simulink model "Battery_charge_discharge_FSBB_DCDC_r2020_batterySelfDesigned"  (R2020a)
settings: Solver=ode23tb  StartTime=0.0  StopTime=1  MaxStep=2.2222222222222224E-7  RelTol=1e-3  EnableMultiTasking=on
undefined symbols (not defined in the file or in its folder): Ion, Lithium, sigbuilder_block
libraries: powerlib x175, dsparch4 x4, simulink x4, electricdrivelib x1, powerlib_meascontrol x1
(part 1 of 2)
settings Model: Creator=Lei  LastModifiedBy=Loki
settings DataIOCC: LimitDataPoints=on  SaveFormat=Array  ReturnWorkspaceOutputs=off
settings OptimizationCC: LifeSpan=inf
settings DebuggingCC: SolverPrmCheckMsg=warning  SFUnexpectedBacktrackingDiag=warning  SFNoUnconditionalDefaultTransitionDiag=warning  SFExecutionAtInitializationDiag=none  ArithmeticOperatorsInVariantConditions=warning
settings HardwareCC: ProdBitPerPointer=32  ProdBitPerSizeT=32  ProdBitPerPtrDiffT=32  ProdLargestAtomicFloat=None  ProdIntDivRoundTo=Undefined  ProdEndianess=Unspecified  ProdWordSize=32  ProdHWDeviceType=32-bit Generic
settings ModelReferenceCC: PropagateSignalLabelsOutOfModel=off
settings SFSimCC: SimUseLocalCustomCode=off  CustomCodeUndefinedFunction=UseInterfaceOnly
settings RTWCC: RTWUseLocalCustomCode=off
settings CodeAppCC: StateflowObjectComments=on
settings GRTTargetCC: TargetLangStandard=C89/C90 (ANSI)
settings ConfigComp: CovMetricSettings=dw  CovSaveCumulativeToWorkspaceVar=on  CovSaveSingleToWorkspaceVar=on  CovExternalEMLEnable=off  CovSFcnEnable=off
settings SimscapeCC: SimscapeNormalizeSystem=off

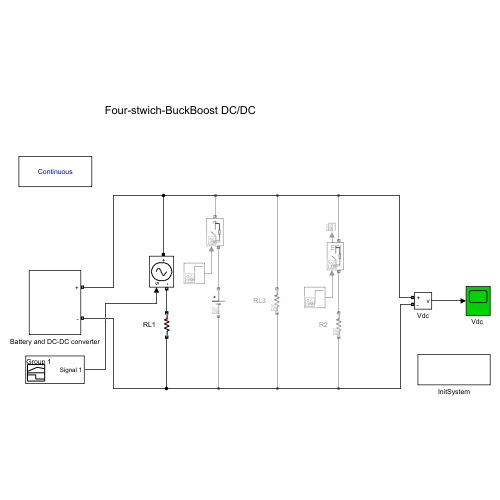
[thumbnail: Simulink's stored preview of the top-level diagram]
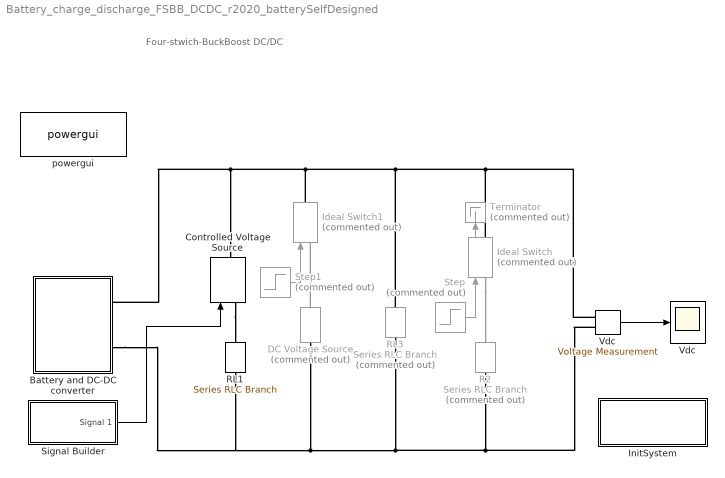
== system Battery_charge_discharge_FSBB_DCDC_r2020_batterySelfDesigned ==
  note: Four-stwich-BuckBoost DC/DC
  Battery and DC-DC converter : Subsystem
  Controlled Voltage Source : powerlib/Electrical Sources/Controlled Voltage Source  Initialize=on  Source_Type=DC  Amplitude=98  Phase=0  Frequency=0  Measurements=None
  DC Voltage Source : powerlib/Electrical Sources/DC Voltage Source  Commented=on  Amplitude=96  Measurements=None
  Ideal Switch : powerlib/Power Electronics/Ideal Switch  Commented=on  Ron=0.001  Lon=0  IC=0  Rs=1e5  Cs=inf  Measurements=on
  Ideal Switch1 : powerlib/Power Electronics/Ideal Switch  Commented=on  Ron=0.001  Lon=0  IC=0  Rs=1e5  Cs=inf  Measurements=off
  InitSystem : Subsystem
      settings: OpenFcn=Battery_charge_discharge_FSBB_param_init
  R2 : powerlib/Elements/Series RLC Branch  Commented=on  LConnTagsString=__new0  RConnTagsString=__new0  BranchType=R  Resistance=6  Inductance=1e-3  SetiL0=off  InitialCurrent=0  Capacitance=1e-6  Setx0=off  InitialVoltage=0  Measurements=None
  RL1 : powerlib/Elements/Series RLC Branch  LConnTagsString=__new0  RConnTagsString=__new0  BranchType=R  Resistance=0.01  Inductance=1e-3  SetiL0=off  InitialCurrent=0  Capacitance=1e-6  Setx0=off  InitialVoltage=0  Measurements=None
  RL3 : powerlib/Elements/Series RLC Branch  Commented=on  LConnTagsString=__new0  RConnTagsString=__new0  BranchType=R  Resistance=3  Inductance=1e-3  SetiL0=off  InitialCurrent=0  Capacitance=1e-6  Setx0=off  InitialVoltage=0  Measurements=None
  Signal Builder : Subsystem  Tag=STV Subsys  LoadFcn=sigbuilder_block('load');  StartFcn=sigbuilder_block('start');  StopFcn=sigbuilder_block('stop');  ClipboardFcn=sigbuilder_block('clipboard');  mask(Sigbuilder block){tuvar=[0:10]}
      mask help: Simulink:masks:SigbuilderBlock_MD
      mask init:
      | if ~strcmp(get_param(bdroot(gcbh),'SimulationStatus'),'stopped') tuvar = sigbuilder_block('maskInit'); end
      settings: CopyFcn=sigbuilder_block('copy');  DeleteFcn=sigbuilder_block('delete');  ModelCloseFcn=sigbuilder_block('modelClose');  PreSaveFcn=sigbuilder_block('preSave');  PauseFcn=sigbuilder_block('pause');  ContinueFcn=sigbuilder_block('continue');  NameChangeFcn=sigbuilder_block('namechange');  OpenFcn=sigbuilder_block('open',[5.4 7.2 1141.2 492.6 ]);  CloseFcn=sigbuilder_block('close');
      mask Display: plot(0, 0, 100, 100,[2, 2, 32, 32, 2], [68, 8, 8, 68, 68],[32, 2], [38, 38], [32, 19, 2],[53, 60, 44], [32, 17, 17, 2],[16, 16, 31, 31]);txt = getActiveGroup(gcbh);text(2, 100, txt,'verticalAlignment', 'top');
  Step : Step  Commented=on  Time=0.3  After=3  SampleTime=0
  Step1 : Step  Commented=on  Time=0.2  SampleTime=0
  Terminator : Terminator  Commented=on
  Vdc : powerlib/Measurements/Voltage Measurement  PhasorSimulation=off  OutputType=Complex  PSBequivalent=0
  "Vdc " : Scope
  powergui : powerlib/powergui  Priority=1  SimulationMode=Continuous  SampleTime=1/45000/100  frequency=60  Iterations=50  frequencyindice=0  Pbase=100e6  ErrMax=1e-4  UnitsV=kV  UnitsW=MW  buscounter=0  FunctionMessages=off  echomessages=off  EnableUseOfTLC=off  CurrentSourceSwitches=off  DisableSnubberDevices=off  DisableRonSwitches=off  DisableVfSwitches=off  DisplayEquations=off  AutomaticDiscreteSolvers=off  SolverType=Tustin/Backward Euler (TBE)  Interpol=off  ExternalGateDelay=off  methode=off  Ts=100  x0status=blocks  SPID=off  SwTol=0  HookPort=off  NonlinearTolerance=1e-4  nMaxIteration=100  ContinueOnMaxIteration=off  RestoreLinks=warning  ResistiveCurrentMeasurement=off  Frange=[0:2:500]  Ylog=off  Xlog=on  ShowGrid=off  save=off  variable=ZData  structure=0  ZoomFFT=off  StartTime=0.0  cycles=1  DisplayStyle=1  fundamental=60  FreqAxis=off  MaxFrequency=1000  frequencyindicesteady=1  RmsSteady=1  display=off
  wires:
  Vdc/1 -> "Vdc "/1
  Step/1 -> Ideal Switch/1
  Ideal Switch/1 -> Terminator/1
  Signal Builder/1(Signal 1) -> Controlled Voltage Source/1
  Step1/1 -> Ideal Switch1/1
  connections:
  Vdc/LConn1 -- Ideal Switch/RConn1 -- Ideal Switch1/RConn1 -- Controlled Voltage Source/RConn1 -- Battery and DC-DC converter/RConn1 -- RL3/LConn1
  Ideal Switch/LConn1 -- R2/LConn1
  Vdc/LConn2 -- R2/RConn1 -- RL1/RConn1 -- Battery and DC-DC converter/RConn2 -- DC Voltage Source/LConn1 -- RL3/RConn1
  Controlled Voltage Source/LConn1 -- RL1/LConn1
  DC Voltage Source/RConn1 -- Ideal Switch1/LConn1

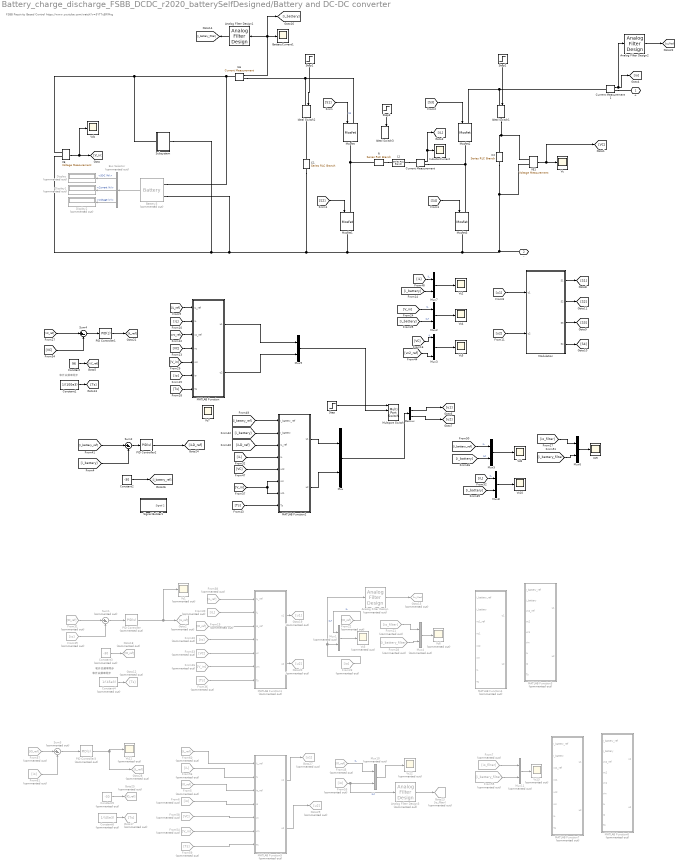
== system Battery_charge_discharge_FSBB_DCDC_r2020_batterySelfDesigned/Battery and DC-DC converter ==
  note: 和开关频率同步
  note: FSBB Passivity Based Control
      | https://www.youtube.com/watch?v=5YT7cERlMrg
  note: 和开关频率同步
  note: 和开关频率同步
  Analog Filter Design : dsparch4/Analog Filter Design  Commented=on  method=Butterworth  filttype=Lowpass  N=1  Wlo=1000  Whi=80  Rp=2  Rs=40
  Analog Filter Design1 : dsparch4/Analog Filter Design  method=Butterworth  filttype=Lowpass  N=1  Wlo=1000  Whi=80  Rp=2  Rs=40
  Analog Filter Design2 : dsparch4/Analog Filter Design  method=Butterworth  filttype=Lowpass  N=1  Wlo=1000  Whi=80  Rp=2  Rs=40
  Analog Filter Design3 : dsparch4/Analog Filter Design  Commented=on  method=Butterworth  filttype=Lowpass  N=1  Wlo=1000  Whi=80  Rp=2  Rs=40
  Battery3 : electricdrivelib/Extra Sources/Battery  Commented=on  BatType=Lithium-Ion  ShowTempParam=off  ThermalPreset=no  ShowAgeParam=off  NomV=102.5  NomQ=10  SOC=50  Batt_Tr=1  PresetModel=on  MaxQ=10  MinV=76.875  FullV=119.3087  Dis_rate=4.3478  R=0.1025  Normal_OP=9.0435  expZone="[110.7395     0.4913043]"  current=[6.5 13 32.5]  Units=Time  Tci=20  NomT=20  T2=-30  MaxQ2=4.8  FullV2=7.1  Normal_OP2=5.655  expZone2="[6.58           1]"  Rca=0.6  ti=2000  Dp=0  Neq0=0  Tsim=1e6  Ta1=25  Qeol=5.4*0.9  Reol=0.013333*1.2  Char_age=[2.3478, 3]  Dis_age=[2.3478, 10]  N1=1500  N2=10500  N3=1000  N4=1400  Ta2=45  N5=950
  BatteryCurrent1 : Scope
  Bus Selector : BusSelector  Commented=on  OutputSignals=SOC (%),Current (A),Voltage (V)
  C1 : powerlib/Elements/Series RLC Branch  LConnTagsString=__new0  RConnTagsString=__new0  BranchType=RC  Resistance=0.001  Inductance=1e-3  SetiL0=off  InitialCurrent=0  Capacitance=1440e-6  Setx0=off  InitialVoltage=80  Measurements=None
  C2 : powerlib/Elements/Series RLC Branch  LConnTagsString=__new0  RConnTagsString=__new0  BranchType=RC  Resistance=0.001  Inductance=1e-3  SetiL0=off  InitialCurrent=0  Capacitance=1440e-6  Setx0=off  InitialVoltage=80  Measurements=None
  Constant : Constant  Value=96
  Constant1 : Constant  Value=1/(100e3)
  Constant2 : Constant  Value=-30
  Constant3 : Constant  Commented=on  Value=-30
  Constant4 : Constant  Commented=on  Value=1/(45e3)
  Constant5 : Constant  Commented=on  Value=-30
  Constant6 : Constant  Commented=on  Value=1/(45e3)
  Current Measurement : powerlib/Measurements/Current Measurement  PhasorSimulation=off  OutputType=Complex  PSBequivalent=0
  Current Measurement1 : powerlib/Measurements/Current Measurement  PhasorSimulation=off  OutputType=Complex  PSBequivalent=0
  Demux : Demux  Outputs=2
  Display : Display  Commented=on
  Display1 : Display  Commented=on
  Display2 : Display  Commented=on
  From{5,19,22,31,45,57} (6 alike) : From  Commented=on  GotoTag=IO_ref
  From{6,20,23,39,53,61} (6 alike) : From  Commented=on  GotoTag=io
  From21 : From  Commented=on  GotoTag=io_filter
  From26 : From  Commented=on  GotoTag=V_in
  From28 : From  Commented=on  GotoTag=i_battery_filter
  From30 : From  Commented=on  GotoTag=iL
  From33 : From  Commented=on  GotoTag=VC
  From36 : From  Commented=on  GotoTag=Ts
  From38 : From  Commented=on  GotoTag=iL_ref
  From54 : From  Commented=on  GotoTag=V_in
  From55 : From  Commented=on  GotoTag=i_battery_filter
  From56 : From  Commented=on  GotoTag=iL
  From58 : From  Commented=on  GotoTag=VC
  From59 : From  Commented=on  GotoTag=Ts
  From60 : From  Commented=on  GotoTag=iL_ref
  From7 : From  Commented=on  GotoTag=io_filter
  Goto12 : Goto  Commented=on  GotoTag=Ts
  Goto15 : Goto  Commented=on  GotoTag=io_filter
  Goto17 : Goto  Commented=on  GotoTag=Ts
  Goto18 : Goto  Commented=on  GotoTag=IO_ref
  Goto19 : Goto  Commented=on  GotoTag=u1
  Goto2 : Goto  Commented=on  GotoTag=iL_ref
  Goto20 : Goto  Commented=on  GotoTag=u2
  Goto23 : Goto  Commented=on  GotoTag=io_filter
  Goto25 : Goto  Commented=on  GotoTag=IO_ref
  Goto27 : Goto  Commented=on  GotoTag=u1
  Goto28 : Goto  Commented=on  GotoTag=iL_ref
  Goto29 : Goto  Commented=on  GotoTag=u2
  IL6 : powerlib/Measurements/Current Measurement  PhasorSimulation=off  OutputType=Complex  PSBequivalent=0
  Ideal Switch1 : powerlib/Power Electronics/Ideal Switch  Ron=1e-6  Lon=0  IC=0  Rs=3  Cs=inf  Measurements=off
  Ideal Switch2 : powerlib/Power Electronics/Ideal Switch  Ron=1e-6  Lon=0  IC=0  Rs=3  Cs=inf  Measurements=off
  Ideal Switch3 : powerlib/Power Electronics/Ideal Switch  Ron=1e-6  Lon=0  IC=0  Rs=3  Cs=inf  Measurements=on
  InductorCurrent : Scope
  L1 : powerlib/Elements/Series RLC Branch  LConnTagsString=__new0  RConnTagsString=__new0  BranchType=L  Resistance=1.0  Inductance=20e-6  SetiL0=off  InitialCurrent=0  Capacitance=1.0  Setx0=off  InitialVoltage=0  Measurements=None
  MATLAB Function : MATLAB Function  TreatAsAtomicUnit=on
  MATLAB Function1 : MATLAB Function  Commented=on  TreatAsAtomicUnit=on
  MATLAB Function2 : MATLAB Function  TreatAsAtomicUnit=on
  MATLAB Function3 : MATLAB Function  Commented=on  TreatAsAtomicUnit=on
  MATLAB Function4 : MATLAB Function  Commented=on  TreatAsAtomicUnit=on
  MATLAB Function5 : MATLAB Function  Commented=on  TreatAsAtomicUnit=on
  MATLAB Function6 : MATLAB Function  Commented=on  TreatAsAtomicUnit=on
  MATLAB Function7 : MATLAB Function  Commented=on  TreatAsAtomicUnit=on
  Modulation : Subsystem
  Mosfet{,1..3} (4 alike) : powerlib/Power Electronics/Mosfet  Ron=0.1  Lon=0  Rd=0.01  Vfd=0  IC=0  Rs=1e5  Cs=inf  Measurements=off
  Multiport Switch : MultiPortSwitch
  Mux{,2,5..9} (7 alike) : Mux  Inputs=2
  Mux{1,4,10..11} (4 alike) : Mux  Commented=on  Inputs=2
  Mux3 : Mux  Inputs=3
  PID Controller : simulink/Continuous/PID Controller  Commented=on  Controller=PID  Form=Parallel  TimeDomain=Continuous-time  UseExternalTs=off  SampleTime=-1  IntegratorMethod=Forward Euler  FilterMethod=Forward Euler  ControllerParametersSource=internal  P=15  I=1000  D=0  N=100  UseFilter=on  TunerSelectOption=Transfer Function Based (PID Tuner App)  InitialConditionSource=internal  InitialConditionForIntegrator=0  InitialConditionForFilter=0  DifferentiatorICPrevScaledInput=0  ExternalReset=none  TrackingMode=off  Kt=1  LimitOutput=off  UpperSaturationLimit=inf  LowerSaturationLimit=-inf  LinearizeAsGain=on  AntiWindupMode=none  Kb=1  POutMin=[]  POutMax=[]  IOutMin=[]  IOutMax=[]  DOutMin=[]  DOutMax=[]  NOutMin=[]  NOutMax=[]  SumOutMin=[]  SumOutMax=[]  SaturationOutMin=[]  SaturationOutMax=[]  PParamMin=[]  PParamMax=[]  IParamMin=[]  IParamMax=[]  DParamMin=[]  DParamMax=[]  NParamMin=[]  NParamMax=[]  KbParamMin=[]  KbParamMax=[]  KtParamMin=[]  KtParamMax=[]  KbOutMin=[]  KbOutMax=[]  KtOutMin=[]  KtOutMax=[]  IntegratorOutMin=[]  IntegratorOutMax=[]  FilterOutMin=[]  FilterOutMax=[]  SumI1OutMin=[]  SumI1OutMax=[]  SumI2OutMin=[]  SumI2OutMax=[]  SumI3OutMin=[]  SumI3OutMax=[]  SumI4OutMin=[]  SumI4OutMax=[]  SumDOutMin=[]  SumDOutMax=[]  DifferentiatorOutMin=[]  DifferentiatorOutMax=[]  FilterDiffOutCoefMin=[]  FilterDiffOutCoefMax=[]  ReciprocalOutMin=[]  ReciprocalOutMax=[]  SumDenOutMin=[]  SumDenOutMax=[]  SumNumOutMin=[]  SumNumOutMax=[]  DivideOutMin=[]  DivideOutMax=[]  UdiffTsProdOutMin=[]  UdiffTsProdOutMax=[]  NTsProdOutMin=[]  NTsProdOutMax=[]  UintegralTsProdOutMin=[]  UintegralTsProdOutMax=[]  UngainTsProdOutMin=[]  UngainTsProdOutMax=[]  IntegratorContinuousStateAttributes=''  IntegratorStateMustResolveToSignalObject=off  IntegratorRTWStateStorageClass=Auto  FilterContinuousStateAttributes=''  FilterStateMustResolveToSignalObject=off  FilterRTWStateStorageClass=Auto  ParallelPVariant=InternalParameters  IdealPVariant=Disabled  IVariant=InternalParameters  DVariant=InternalParameters  IntegratorVariant=Continuous  SatVariant=Disabled  AWVariant=Passthrough  PCopyVariant=Disabled  TRVariant=Disabled  FdbkBlocksVariant=Forward  IdealPFdbkVariant=Disabled  SatFdbkVariant=Disabled  DerivativeFilterVariant=ContFilter  NVariant=InternalParameters  NCopyVariant=Disabled  FilterICVariant=InternalICsFilter  IntegratorICVariant=InternalICs  ExternalResetVariant=Disabled  TRSumVariant=Passthrough  SumFdbkVariant=Disabled  SumVariant=Sum_PID  TsampFilterVariant=InternalTs  TsampNgainVariant=Passthrough  TsampIntegralVariant=Passthrough
  PID Controller1 : simulink/Continuous/PID Controller  Controller=PID  Form=Parallel  TimeDomain=Discrete-time  UseExternalTs=off  SampleTime=-1  IntegratorMethod=Forward Euler  FilterMethod=Forward Euler  ControllerParametersSource=internal  P=15  I=1000  D=0  N=100  UseFilter=on  TunerSelectOption=Transfer Function Based (PID Tuner App)  InitialConditionSource=internal  InitialConditionForIntegrator=0  InitialConditionForFilter=0  DifferentiatorICPrevScaledInput=0  ExternalReset=none  TrackingMode=off  Kt=1  LimitOutput=off  UpperSaturationLimit=inf  LowerSaturationLimit=-inf  LinearizeAsGain=on  AntiWindupMode=none  Kb=1  POutMin=[]  POutMax=[]  IOutMin=[]  IOutMax=[]  DOutMin=[]  DOutMax=[]  NOutMin=[]  NOutMax=[]  SumOutMin=[]  SumOutMax=[]  SaturationOutMin=[]  SaturationOutMax=[]  PParamMin=[]  PParamMax=[]  IParamMin=[]  IParamMax=[]  DParamMin=[]  DParamMax=[]  NParamMin=[]  NParamMax=[]  KbParamMin=[]  KbParamMax=[]  KtParamMin=[]  KtParamMax=[]  KbOutMin=[]  KbOutMax=[]  KtOutMin=[]  KtOutMax=[]  IntegratorOutMin=[]  IntegratorOutMax=[]  FilterOutMin=[]  FilterOutMax=[]  SumI1OutMin=[]  SumI1OutMax=[]  SumI2OutMin=[]  SumI2OutMax=[]  SumI3OutMin=[]  SumI3OutMax=[]  SumI4OutMin=[]  SumI4OutMax=[]  SumDOutMin=[]  SumDOutMax=[]  DifferentiatorOutMin=[]  DifferentiatorOutMax=[]  FilterDiffOutCoefMin=[]  FilterDiffOutCoefMax=[]  ReciprocalOutMin=[]  ReciprocalOutMax=[]  SumDenOutMin=[]  SumDenOutMax=[]  SumNumOutMin=[]  SumNumOutMax=[]  DivideOutMin=[]  DivideOutMax=[]  UdiffTsProdOutMin=[]  UdiffTsProdOutMax=[]  NTsProdOutMin=[]  NTsProdOutMax=[]  UintegralTsProdOutMin=[]  UintegralTsProdOutMax=[]  UngainTsProdOutMin=[]  UngainTsProdOutMax=[]  IntegratorContinuousStateAttributes=''  IntegratorStateMustResolveToSignalObject=off  IntegratorRTWStateStorageClass=Auto  FilterContinuousStateAttributes=''  FilterStateMustResolveToSignalObject=off  FilterRTWStateStorageClass=Auto  ParallelPVariant=InternalParameters  IdealPVariant=Disabled  IVariant=InternalParameters  DVariant=InternalParameters  IntegratorVariant=Discrete  SatVariant=Disabled  AWVariant=Passthrough  PCopyVariant=Disabled  TRVariant=Disabled  FdbkBlocksVariant=Forward  IdealPFdbkVariant=Disabled  SatFdbkVariant=Disabled  DerivativeFilterVariant=ForwardEulerFilter  NVariant=InternalParameters  NCopyVariant=Disabled  FilterICVariant=InternalICsFilter  IntegratorICVariant=InternalICs  ExternalResetVariant=Disabled  TRSumVariant=Passthrough  SumFdbkVariant=Disabled  SumVariant=Sum_PID  TsampFilterVariant=InternalTs  TsampNgainVariant=Passthrough  TsampIntegralVariant=Passthrough
  PID Controller2 : simulink/Continuous/PID Controller  Controller=PID  Form=Parallel  TimeDomain=Continuous-time  UseExternalTs=off  SampleTime=-1  IntegratorMethod=Forward Euler  FilterMethod=Forward Euler  ControllerParametersSource=internal  P=15  I=2000  D=0  N=100  UseFilter=on  TunerSelectOption=Transfer Function Based (PID Tuner App)  InitialConditionSource=internal  InitialConditionForIntegrator=0  InitialConditionForFilter=0  DifferentiatorICPrevScaledInput=0  ExternalReset=none  TrackingMode=off  Kt=1  LimitOutput=off  UpperSaturationLimit=100  LowerSaturationLimit=-100  LinearizeAsGain=off  AntiWindupMode=none  Kb=1  POutMin=[]  POutMax=[]  IOutMin=[]  IOutMax=[]  DOutMin=[]  DOutMax=[]  NOutMin=[]  NOutMax=[]  SumOutMin=[]  SumOutMax=[]  SaturationOutMin=[]  SaturationOutMax=[]  PParamMin=[]  PParamMax=[]  IParamMin=[]  IParamMax=[]  DParamMin=[]  DParamMax=[]  NParamMin=[]  NParamMax=[]  KbParamMin=[]  KbParamMax=[]  KtParamMin=[]  KtParamMax=[]  KbOutMin=[]  KbOutMax=[]  KtOutMin=[]  KtOutMax=[]  IntegratorOutMin=[]  IntegratorOutMax=[]  FilterOutMin=[]  FilterOutMax=[]  SumI1OutMin=[]  SumI1OutMax=[]  SumI2OutMin=[]  SumI2OutMax=[]  SumI3OutMin=[]  SumI3OutMax=[]  SumI4OutMin=[]  SumI4OutMax=[]  SumDOutMin=[]  SumDOutMax=[]  DifferentiatorOutMin=[]  DifferentiatorOutMax=[]  FilterDiffOutCoefMin=[]  FilterDiffOutCoefMax=[]  ReciprocalOutMin=[]  ReciprocalOutMax=[]  SumDenOutMin=[]  SumDenOutMax=[]  SumNumOutMin=[]  SumNumOutMax=[]  DivideOutMin=[]  DivideOutMax=[]  UdiffTsProdOutMin=[]  UdiffTsProdOutMax=[]  NTsProdOutMin=[]  NTsProdOutMax=[]  UintegralTsProdOutMin=[]  UintegralTsProdOutMax=[]  UngainTsProdOutMin=[]  UngainTsProdOutMax=[]  IntegratorContinuousStateAttributes=''  IntegratorStateMustResolveToSignalObject=off  IntegratorRTWStateStorageClass=Auto  FilterContinuousStateAttributes=''  FilterStateMustResolveToSignalObject=off  FilterRTWStateStorageClass=Auto  ParallelPVariant=InternalParameters  IdealPVariant=Disabled  IVariant=InternalParameters  DVariant=InternalParameters  IntegratorVariant=Continuous  SatVariant=Disabled  AWVariant=Passthrough  PCopyVariant=Disabled  TRVariant=Disabled  FdbkBlocksVariant=Forward  IdealPFdbkVariant=Disabled  SatFdbkVariant=Disabled  DerivativeFilterVariant=ContFilter  NVariant=InternalParameters  NCopyVariant=Disabled  FilterICVariant=InternalICsFilter  IntegratorICVariant=InternalICs  ExternalResetVariant=Disabled  TRSumVariant=Passthrough  SumFdbkVariant=Disabled  SumVariant=Sum_PID  TsampFilterVariant=InternalTs  TsampNgainVariant=Passthrough  TsampIntegralVariant=Passthrough
  PID Controller3 : simulink/Continuous/PID Controller  Commented=on  Controller=PID  Form=Parallel  TimeDomain=Continuous-time  UseExternalTs=off  SampleTime=-1  IntegratorMethod=Forward Euler  FilterMethod=Forward Euler  ControllerParametersSource=internal  P=15  I=1000  D=0  N=100  UseFilter=on  TunerSelectOption=Transfer Function Based (PID Tuner App)  InitialConditionSource=internal  InitialConditionForIntegrator=0  InitialConditionForFilter=0  DifferentiatorICPrevScaledInput=0  ExternalReset=none  TrackingMode=off  Kt=1  LimitOutput=off  UpperSaturationLimit=inf  LowerSaturationLimit=-inf  LinearizeAsGain=on  AntiWindupMode=none  Kb=1  POutMin=[]  POutMax=[]  IOutMin=[]  IOutMax=[]  DOutMin=[]  DOutMax=[]  NOutMin=[]  NOutMax=[]  SumOutMin=[]  SumOutMax=[]  SaturationOutMin=[]  SaturationOutMax=[]  PParamMin=[]  PParamMax=[]  IParamMin=[]  IParamMax=[]  DParamMin=[]  DParamMax=[]  NParamMin=[]  NParamMax=[]  KbParamMin=[]  KbParamMax=[]  KtParamMin=[]  KtParamMax=[]  KbOutMin=[]  KbOutMax=[]  KtOutMin=[]  KtOutMax=[]  IntegratorOutMin=[]  IntegratorOutMax=[]  FilterOutMin=[]  FilterOutMax=[]  SumI1OutMin=[]  SumI1OutMax=[]  SumI2OutMin=[]  SumI2OutMax=[]  SumI3OutMin=[]  SumI3OutMax=[]  SumI4OutMin=[]  SumI4OutMax=[]  SumDOutMin=[]  SumDOutMax=[]  DifferentiatorOutMin=[]  DifferentiatorOutMax=[]  FilterDiffOutCoefMin=[]  FilterDiffOutCoefMax=[]  ReciprocalOutMin=[]  ReciprocalOutMax=[]  SumDenOutMin=[]  SumDenOutMax=[]  SumNumOutMin=[]  SumNumOutMax=[]  DivideOutMin=[]  DivideOutMax=[]  UdiffTsProdOutMin=[]  UdiffTsProdOutMax=[]  NTsProdOutMin=[]  NTsProdOutMax=[]  UintegralTsProdOutMin=[]  UintegralTsProdOutMax=[]  UngainTsProdOutMin=[]  UngainTsProdOutMax=[]  IntegratorContinuousStateAttributes=''  IntegratorStateMustResolveToSignalObject=off  IntegratorRTWStateStorageClass=Auto  FilterContinuousStateAttributes=''  FilterStateMustResolveToSignalObject=off  FilterRTWStateStorageClass=Auto  ParallelPVariant=InternalParameters  IdealPVariant=Disabled  IVariant=InternalParameters  DVariant=InternalParameters  IntegratorVariant=Continuous  SatVariant=Disabled  AWVariant=Passthrough  PCopyVariant=Disabled  TRVariant=Disabled  FdbkBlocksVariant=Forward  IdealPFdbkVariant=Disabled  SatFdbkVariant=Disabled  DerivativeFilterVariant=ContFilter  NVariant=InternalParameters  NCopyVariant=Disabled  FilterICVariant=InternalICsFilter  IntegratorICVariant=InternalICs  ExternalResetVariant=Disabled  TRSumVariant=Passthrough  SumFdbkVariant=Disabled  SumVariant=Sum_PID  TsampFilterVariant=InternalTs  TsampNgainVariant=Passthrough  TsampIntegralVariant=Passthrough
  R : powerlib/Elements/Series RLC Branch  LConnTagsString=__new0  RConnTagsString=__new0  BranchType=R  Resistance=0.004  Inductance=1e-3  SetiL0=off  InitialCurrent=0  Capacitance=1e-3  Setx0=off  InitialVoltage=80  Measurements=None
  Signal Builder1 : Subsystem  Tag=STV Subsys  LoadFcn=sigbuilder_block('load');  StartFcn=sigbuilder_block('start');  StopFcn=sigbuilder_block('stop');  ClipboardFcn=sigbuilder_block('clipboard');  mask(Sigbuilder block){tuvar=[0:10]}
      mask help: Simulink:masks:SigbuilderBlock_MD
      mask init:
      | if ~strcmp(get_param(bdroot(gcbh),'SimulationStatus'),'stopped') tuvar = sigbuilder_block('maskInit'); end
      settings: CopyFcn=sigbuilder_block('copy');  DeleteFcn=sigbuilder_block('delete');  ModelCloseFcn=sigbuilder_block('modelClose');  PreSaveFcn=sigbuilder_block('preSave');  PauseFcn=sigbuilder_block('pause');  ContinueFcn=sigbuilder_block('continue');  NameChangeFcn=sigbuilder_block('namechange');  OpenFcn=sigbuilder_block('open',[162.6 186.6 550.8 400.2 ]);  CloseFcn=sigbuilder_block('close');
      mask Display: plot(0, 0, 100, 100,[2, 2, 32, 32, 2], [68, 8, 8, 68, 68],[32, 2], [38, 38], [32, 19, 2],[53, 60, 44], [32, 17, 17, 2],[16, 16, 31, 31]);txt = getActiveGroup(gcbh);text(2, 100, txt,'verticalAlignment', 'top');
  Step : Step  Time=0.2  Before=2  After=2  SampleTime=0
  Step1 : Step  Time=0.02  SampleTime=0
  Step2 : Step  Time=0.02  SampleTime=0
  Step3 : Step  Time=0.02  SampleTime=0
  Subsystem : Subsystem
  Sum1 : Sum  Commented=on  Inputs=|+-
  Sum2 : Sum  Inputs=|+-
  Sum3 : Sum  Commented=on  Inputs=|+-
  Sum4 : Sum  Inputs=|+-
  VE : powerlib/Measurements/Voltage Measurement  PhasorSimulation=off  OutputType=Complex  PSBequivalent=0
  VE1 : powerlib/Measurements/Voltage Measurement  PhasorSimulation=off  OutputType=Complex  PSBequivalent=0
  Vc{,2,4..5,7..10} (8 alike) : Scope
  Vc{1,3,6,11..13} (6 alike) : Scope  Commented=on
  "Vdc " : Scope
  + : PMIOPort  Tag=PMCPort  Side=Right
  - : PMIOPort  Tag=PMCPort  Port=2  Side=Right
  wires:
  VE/1 -> "Vdc "/1, [V_in]
  IL6/1 -> [i_battery], Analog Filter Design1/1, BatteryCurrent1/1
  Battery3/1 -> Bus Selector/1
  [S2] -> Mosfet1/1
  [S1] -> Mosfet/1  "S1"
  Current Measurement/1 -> [iL], InductorCurrent/1
  [S3] -> Mosfet2/1
  [S4] -> Mosfet3/1
  [iL_ref] -> MATLAB Function/1(iL_ref)
  [iL] -> MATLAB Function/2(iL)
  Constant/1 -> [VC_ref]
  [VC_ref] -> MATLAB Function/3(vc_ref)
  [VC] -> MATLAB Function/4(vc)
  [V_in] -> MATLAB Function/5(vin)
  [Ts] -> MATLAB Function/7(Ts)
  [io] -> MATLAB Function/6(io)
  [u1] -> Modulation/1(u1)
  [u2] -> Modulation/2(u2)
  Modulation/1(S1) -> [S1]
  Modulation/3(S3) -> [S3]
  Modulation/4(S4) -> [S4]
  Modulation/2(S2) -> [S2]
  Constant1/1 -> [Ts]
  VE1/1 -> [VC], Vc/1
  From39/1 -> Sum1/2
  From31/1 -> Sum1/1
  From38/1 -> MATLAB Function1/1(iL_ref)
  Constant4/1 -> Goto12/1
  From30/1 -> MATLAB Function1/2(iL)
  Sum1/1 -> PID Controller/1
  Constant3/1 -> Goto18/1
  From19/1 -> MATLAB Function1/3(io_ref)
  From36/1 -> MATLAB Function1/7(Ts)
  From33/1 -> MATLAB Function1/5(vc)
  From20/1 -> MATLAB Function1/4(io)
  From26/1 -> MATLAB Function1/6(vin)
  Bus Selector/1 -> Display/1  "<SOC (%)>"
  Bus Selector/2 -> Display1/1  "<Current (A)>"
  Bus Selector/3 -> Display2/1  "<Voltage (V)>"
  MATLAB Function1/1(u1) -> Goto19/1
  MATLAB Function1/2(u2) -> Goto20/1
  MATLAB Function/2(u2) -> Mux9/2
  MATLAB Function/1(u1) -> Mux9/1
  PID Controller1/1 -> [iL_ref]
  Sum4/1 -> PID Controller1/1
  [VC] -> Sum4/2
  [VC_ref] -> Sum4/1
  PID Controller/1 -> Vc1/1, Goto2/1
  From23/1 -> Analog Filter Design/1, Mux1/2  "iL*"
  Mux1/1 -> Vc3/1
  From22/1 -> Mux1/1  "iL"
  [V_in] -> Mux2/1  "iL"
  [iL] -> Mux7/1  "iL"
  [i_battery] -> Mux7/2
  [i_battery] -> Mux2/2  "iL*"
  Mux7/1 -> Vc2/1
  Mux2/1 -> Vc4/1
  Mux3/1 -> Vc5/1
  [vc2_ref] -> Mux3/3
  [VC] -> Mux3/1  "iL"
  Step2/1 -> Ideal Switch1/1
  Analog Filter Design/1 -> Goto15/1
  Analog Filter Design1/1 -> [i_battery_filter]
  Mux4/1 -> Vc6/1
  From28/1 -> Mux4/2
  From21/1 -> Mux4/1
  MATLAB Function2/2(u2) -> Mux/2
  MATLAB Function2/1(u1) -> Mux/1
  Sum2/1 -> PID Controller2/1
  [i_battery_ref] -> Sum2/1
  [i_battery] -> Sum2/2
  [i_battery_ref] -> MATLAB Function2/1(i_battery_ref)
  [i_battery] -> MATLAB Function2/2(i_battery)
  [io_filter] -> Mux6/1
  Mux6/1 -> Vc9/1
  Analog Filter Design2/1 -> [io_filter]
  [i_battery_filter] -> Mux6/2
  Mux5/1 -> Vc8/1
  [i_battery_ref] -> Mux5/1  "iL"
  [i_battery] -> Mux5/2  "iL*"
  Current Measurement1/1 -> Analog Filter Design2/1, [io]
  [Ts] -> MATLAB Function2/8(Ts)
  [iLD_ref] -> MATLAB Function2/3(iL_ref)
  Mux8/1 -> Vc10/1
  [iL] -> Mux8/1  "iL"
  [i_battery] -> Mux8/2
  Mux9/1 -> Multiport Switch/2
  Demux/1 -> [u1]
  Demux/2 -> [u2]
  [V_in] -> MATLAB Function2/6(vin), MATLAB Function2/7(vc1)
  [iL] -> MATLAB Function2/4(iL)
  [VC] -> MATLAB Function2/5(vc2)
  PID Controller2/1 -> [iLD_ref]
  Step1/1 -> Ideal Switch2/1
  Step3/1 -> Ideal Switch3/1
  Step/1 -> Multiport Switch/1
  Constant2/1 -> [i_battery_ref]
  From7/1 -> Mux11/1
  From55/1 -> Mux11/2
  Mux11/1 -> Vc13/1
  Analog Filter Design3/1 -> Goto23/1
  From45/1 -> Mux10/1  "iL"
  Mux10/1 -> Vc12/1
  From53/1 -> Mux10/2, Analog Filter Design3/1  "iL*"
  PID Controller3/1 -> Vc11/1, Goto28/1
  MATLAB Function5/2(u2) -> Goto29/1
  MATLAB Function5/1(u1) -> Goto27/1
  From54/1 -> MATLAB Function5/6(vin)
  From6/1 -> MATLAB Function5/4(io)
  From58/1 -> MATLAB Function5/5(vc)
  From59/1 -> MATLAB Function5/7(Ts)
  From5/1 -> MATLAB Function5/3(io_ref)
  Constant5/1 -> Goto25/1
  Sum3/1 -> PID Controller3/1
  From56/1 -> MATLAB Function5/2(iL)
  Constant6/1 -> Goto17/1
  From60/1 -> MATLAB Function5/1(iL_ref)
  From57/1 -> Sum3/1
  From61/1 -> Sum3/2
  Mux/1 -> Demux/1
  connections:
  C2/RConn1 -- VE1/LConn2 -- -/RConn1 -- Mosfet3/RConn1 -- Subsystem/RConn1 -- VE/LConn2 -- Battery3/LConn2 -- C1/RConn1 -- Mosfet1/RConn1
  VE/LConn1 -- Battery3/LConn1 -- IL6/LConn1 -- Subsystem/LConn1
  C1/LConn1 -- Ideal Switch2/RConn1
  Mosfet1/LConn1 -- R/RConn1 -- Mosfet/RConn1
  Current Measurement/RConn1 -- Mosfet3/LConn1 -- Mosfet2/RConn1
  L1/RConn1 -- Current Measurement/LConn1
  R/LConn1 -- L1/LConn1
  Current Measurement1/RConn1 -- +/RConn1
  Mosfet2/LConn1 -- Current Measurement1/LConn1 -- Ideal Switch1/LConn1
  C2/LConn1 -- Ideal Switch1/RConn1 -- VE1/LConn1
  Ideal Switch2/LConn1 -- Mosfet/LConn1 -- IL6/RConn1

== system Battery_charge_discharge_FSBB_DCDC_r2020_batterySelfDesigned/InitSystem ==

== system Battery_charge_discharge_FSBB_DCDC_r2020_batterySelfDesigned/Signal Builder ==
  Demux : Demux  Tag=STV Demux  Outputs=1
      settings: DisplayOption=none
  FromWs : FromWorkspace  Tag=STV FromWs  VariableName=tuvar
      SigBuilderData=|
      | common.afterFinalStr = 'Extrapolate'
      | common.sampleTime = 0
      | dataSet.timeRange = [0 5]
      | dataSet.name = 'Group 1'
      | sbobj.Groups.Name = 'Group 1'
      | sbobj.Groups.Signals.Name = 'Signal 1'
      | sbobj.Groups.Signals.XData = [0 0.3 0.4 0.41 0.41 0.42 0.6 0.61 1 2 2 5]
      | sbobj.Groups.Signals.YData = [97.2 97.9 100 120.2 120 110 110 81.2 83.3 81.4 81.3 79.4]
      | sbobj.Groups.TimeRange = [0 5]
  Signal 1 : Outport  Tag=STV Outport
  wires:
  Demux/1 -> Signal 1/1
  FromWs/1 -> Demux/1

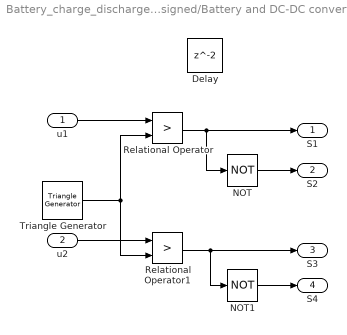
== system Battery_charge_discharge_FSBB_DCDC_r2020_batterySelfDesigned/Battery and DC-DC converter/Modulation ==
  u1 : Inport
  u2 : Inport  Port=2
  Delay : Delay
  NOT : Logic  Operator=NOT  AllPortsSameDT=off  OutDataTypeStr=boolean
  NOT1 : Logic  Operator=NOT  AllPortsSameDT=off  OutDataTypeStr=boolean
  Relational Operator : RelationalOperator  Operator=>  OutDataTypeStr=boolean  RndMeth=Simplest
  Relational Operator1 : RelationalOperator  Operator=>  OutDataTypeStr=boolean  RndMeth=Simplest
  Triangle Generator : powerlib_meascontrol/Pulse & Signal Generators/Triangle Generator  Freq=100e3  Phase=0  Ts=0
  S1 : Outport
  S2 : Outport  Port=2
  S3 : Outport  Port=3
  S4 : Outport  Port=4
  wires:
  u1/1 -> Relational Operator/1
  Triangle Generator/1 -> Relational Operator1/2, Relational Operator/2
  u2/1 -> Relational Operator1/1
  Relational Operator/1 -> NOT/1, S1/1
  NOT/1 -> S2/1
  Relational Operator1/1 -> NOT1/1, S3/1
  NOT1/1 -> S4/1

== system Battery_charge_discharge_FSBB_DCDC_r2020_batterySelfDesigned/Battery and DC-DC converter/Signal Builder1 ==
  Demux : Demux  Tag=STV Demux  Outputs=1
      settings: DisplayOption=none
  FromWs : FromWorkspace  Tag=STV FromWs  VariableName=tuvar
      SigBuilderData=|
      | common.afterFinalStr = 'Extrapolate'
      | common.sampleTime = 0
      | dataSet.timeRange = [0 10]
      | dataSet.name = 'Group 1'
      | sbobj.Groups.Name = 'Group 1'
      | sbobj.Groups.Signals.Name = 'Signal 2'
      | sbobj.Groups.Signals.XData = [0 0.2 0.4 1 5 10]
      | sbobj.Groups.Signals.YData = [0 0 -30 -30 1 1]
  Signal 2 : Outport  Tag=STV Outport
  wires:
  FromWs/1 -> Demux/1
  Demux/1 -> Signal 2/1

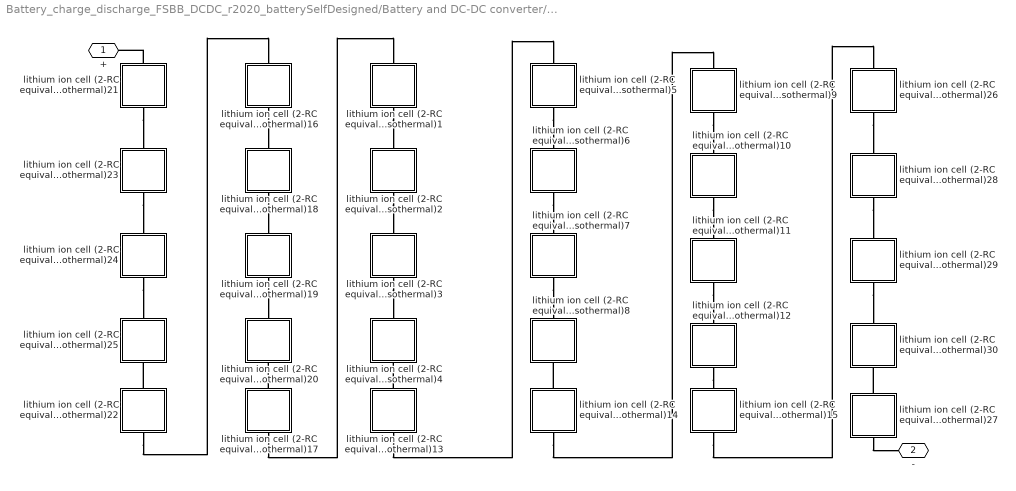
== system Battery_charge_discharge_FSBB_DCDC_r2020_batterySelfDesigned/Battery and DC-DC converter/Subsystem ==
  "lithium ion cell (2-RC equivalent circuit model, isothermal)1" : Subsystem
  "lithium ion cell (2-RC equivalent circuit model, isothermal)10" : Subsystem
  "lithium ion cell (2-RC equivalent circuit model, isothermal)11" : Subsystem
  "lithium ion cell (2-RC equivalent circuit model, isothermal)12" : Subsystem
  "lithium ion cell (2-RC equivalent circuit model, isothermal)13" : Subsystem
  "lithium ion cell (2-RC equivalent circuit model, isothermal)14" : Subsystem
  "lithium ion cell (2-RC equivalent circuit model, isothermal)15" : Subsystem
  "lithium ion cell (2-RC equivalent circuit model, isothermal)16" : Subsystem
  "lithium ion cell (2-RC equivalent circuit model, isothermal)17" : Subsystem
  "lithium ion cell (2-RC equivalent circuit model, isothermal)18" : Subsystem
  "lithium ion cell (2-RC equivalent circuit model, isothermal)19" : Subsystem
  "lithium ion cell (2-RC equivalent circuit model, isothermal)2" : Subsystem
  "lithium ion cell (2-RC equivalent circuit model, isothermal)20" : Subsystem
  "lithium ion cell (2-RC equivalent circuit model, isothermal)21" : Subsystem
  "lithium ion cell (2-RC equivalent circuit model, isothermal)22" : Subsystem
  "lithium ion cell (2-RC equivalent circuit model, isothermal)23" : Subsystem
  "lithium ion cell (2-RC equivalent circuit model, isothermal)24" : Subsystem
  "lithium ion cell (2-RC equivalent circuit model, isothermal)25" : Subsystem
  "lithium ion cell (2-RC equivalent circuit model, isothermal)26" : Subsystem
  "lithium ion cell (2-RC equivalent circuit model, isothermal)27" : Subsystem
  "lithium ion cell (2-RC equivalent circuit model, isothermal)28" : Subsystem
  "lithium ion cell (2-RC equivalent circuit model, isothermal)29" : Subsystem
  "lithium ion cell (2-RC equivalent circuit model, isothermal)3" : Subsystem
  "lithium ion cell (2-RC equivalent circuit model, isothermal)30" : Subsystem
  "lithium ion cell (2-RC equivalent circuit model, isothermal)4" : Subsystem
  "lithium ion cell (2-RC equivalent circuit model, isothermal)5" : Subsystem
  "lithium ion cell (2-RC equivalent circuit model, isothermal)6" : Subsystem
  "lithium ion cell (2-RC equivalent circuit model, isothermal)7" : Subsystem
  "lithium ion cell (2-RC equivalent circuit model, isothermal)8" : Subsystem
  "lithium ion cell (2-RC equivalent circuit model, isothermal)9" : Subsystem
  + : PMIOPort  Side=Left
  - : PMIOPort  Port=2  Side=Right
  connections:
  "lithium ion cell (2-RC equivalent circuit model, isothermal)14"/RConn1 -- "lithium ion cell (2-RC equivalent circuit model, isothermal)9"/LConn1
  "lithium ion cell (2-RC equivalent circuit model, isothermal)11"/RConn1 -- "lithium ion cell (2-RC equivalent circuit model, isothermal)12"/LConn1
  "lithium ion cell (2-RC equivalent circuit model, isothermal)3"/RConn1 -- "lithium ion cell (2-RC equivalent circuit model, isothermal)4"/LConn1
  "lithium ion cell (2-RC equivalent circuit model, isothermal)27"/RConn1 -- -/RConn1
  "lithium ion cell (2-RC equivalent circuit model, isothermal)17"/RConn1 -- "lithium ion cell (2-RC equivalent circuit model, isothermal)1"/LConn1
  "lithium ion cell (2-RC equivalent circuit model, isothermal)17"/LConn1 -- "lithium ion cell (2-RC equivalent circuit model, isothermal)20"/RConn1
  "lithium ion cell (2-RC equivalent circuit model, isothermal)13"/RConn1 -- "lithium ion cell (2-RC equivalent circuit model, isothermal)5"/LConn1
  "lithium ion cell (2-RC equivalent circuit model, isothermal)13"/LConn1 -- "lithium ion cell (2-RC equivalent circuit model, isothermal)4"/RConn1
  "lithium ion cell (2-RC equivalent circuit model, isothermal)2"/RConn1 -- "lithium ion cell (2-RC equivalent circuit model, isothermal)3"/LConn1
  "lithium ion cell (2-RC equivalent circuit model, isothermal)14"/LConn1 -- "lithium ion cell (2-RC equivalent circuit model, isothermal)8"/RConn1
  "lithium ion cell (2-RC equivalent circuit model, isothermal)26"/RConn1 -- "lithium ion cell (2-RC equivalent circuit model, isothermal)28"/LConn1
  "lithium ion cell (2-RC equivalent circuit model, isothermal)23"/RConn1 -- "lithium ion cell (2-RC equivalent circuit model, isothermal)24"/LConn1
  "lithium ion cell (2-RC equivalent circuit model, isothermal)19"/RConn1 -- "lithium ion cell (2-RC equivalent circuit model, isothermal)20"/LConn1
  "lithium ion cell (2-RC equivalent circuit model, isothermal)9"/RConn1 -- "lithium ion cell (2-RC equivalent circuit model, isothermal)10"/LConn1
  "lithium ion cell (2-RC equivalent circuit model, isothermal)15"/RConn1 -- "lithium ion cell (2-RC equivalent circuit model, isothermal)26"/LConn1
  "lithium ion cell (2-RC equivalent circuit model, isothermal)18"/RConn1 -- "lithium ion cell (2-RC equivalent circuit model, isothermal)19"/LConn1
  "lithium ion cell (2-RC equivalent circuit model, isothermal)10"/RConn1 -- "lithium ion cell (2-RC equivalent circuit model, isothermal)11"/LConn1
  "lithium ion cell (2-RC equivalent circuit model, isothermal)22"/RConn1 -- "lithium ion cell (2-RC equivalent circuit model, isothermal)16"/LConn1
  "lithium ion cell (2-RC equivalent circuit model, isothermal)1"/RConn1 -- "lithium ion cell (2-RC equivalent circuit model, isothermal)2"/LConn1
  "lithium ion cell (2-RC equivalent circuit model, isothermal)28"/RConn1 -- "lithium ion cell (2-RC equivalent circuit model, isothermal)29"/LConn1
  "lithium ion cell (2-RC equivalent circuit model, isothermal)29"/RConn1 -- "lithium ion cell (2-RC equivalent circuit model, isothermal)30"/LConn1
  "lithium ion cell (2-RC equivalent circuit model, isothermal)27"/LConn1 -- "lithium ion cell (2-RC equivalent circuit model, isothermal)30"/RConn1
  "lithium ion cell (2-RC equivalent circuit model, isothermal)7"/RConn1 -- "lithium ion cell (2-RC equivalent circuit model, isothermal)8"/LConn1
  "lithium ion cell (2-RC equivalent circuit model, isothermal)5"/RConn1 -- "lithium ion cell (2-RC equivalent circuit model, isothermal)6"/LConn1
  "lithium ion cell (2-RC equivalent circuit model, isothermal)6"/RConn1 -- "lithium ion cell (2-RC equivalent circuit model, isothermal)7"/LConn1
  "lithium ion cell (2-RC equivalent circuit model, isothermal)16"/RConn1 -- "lithium ion cell (2-RC equivalent circuit model, isothermal)18"/LConn1
  "lithium ion cell (2-RC equivalent circuit model, isothermal)24"/RConn1 -- "lithium ion cell (2-RC equivalent circuit model, isothermal)25"/LConn1
  "lithium ion cell (2-RC equivalent circuit model, isothermal)21"/RConn1 -- "lithium ion cell (2-RC equivalent circuit model, isothermal)23"/LConn1
  "lithium ion cell (2-RC equivalent circuit model, isothermal)22"/LConn1 -- "lithium ion cell (2-RC equivalent circuit model, isothermal)25"/RConn1
  "lithium ion cell (2-RC equivalent circuit model, isothermal)12"/RConn1 -- "lithium ion cell (2-RC equivalent circuit model, isothermal)15"/LConn1
  "lithium ion cell (2-RC equivalent circuit model, isothermal)21"/LConn1 -- +/RConn1

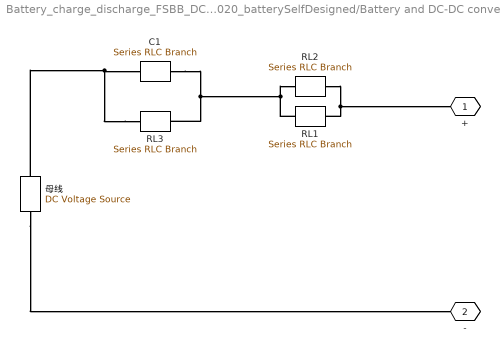
== system Battery_charge_discharge_FSBB_DCDC_r2020_batterySelfDesigned/Battery and DC-DC converter/Subsystem/lithium ion cell (2-RC equivalent circuit model, isothermal)1 ==
  C1 : powerlib/Elements/Series RLC Branch  LConnTagsString=__new0  RConnTagsString=__new0  BranchType=C  Resistance=5  Inductance=1e-3  SetiL0=off  InitialCurrent=0  Capacitance=193  Setx0=off  InitialVoltage=80  Measurements=None
  RL1 : powerlib/Elements/Series RLC Branch  LConnTagsString=__new0  RConnTagsString=__new0  BranchType=R  Resistance=0.86e-3  Inductance=1e-3  SetiL0=off  InitialCurrent=0  Capacitance=1e-6  Setx0=off  InitialVoltage=0  Measurements=None
  RL2 : powerlib/Elements/Series RLC Branch  LConnTagsString=__new0  RConnTagsString=__new0  BranchType=R  Resistance=0.78e-3  Inductance=1e-3  SetiL0=off  InitialCurrent=0  Capacitance=1e-6  Setx0=off  InitialVoltage=0  Measurements=None
  RL3 : powerlib/Elements/Series RLC Branch  LConnTagsString=__new0  RConnTagsString=__new0  BranchType=R  Resistance=0.78e-3  Inductance=1e-3  SetiL0=off  InitialCurrent=0  Capacitance=1e-6  Setx0=off  InitialVoltage=0  Measurements=None
  "母线  " : powerlib/Electrical Sources/DC Voltage Source  Amplitude=3.2  Measurements=None
  + : PMIOPort  Tag=PMCPort  Side=Left
  - : PMIOPort  Tag=PMCPort  Port=2  Side=Right
  connections:
  RL3/LConn1 -- "母线  "/RConn1 -- C1/LConn1
  "母线  "/LConn1 -- -/RConn1
  RL2/RConn1 -- RL1/RConn1 -- +/RConn1
  RL2/LConn1 -- RL1/LConn1 -- RL3/RConn1 -- C1/RConn1

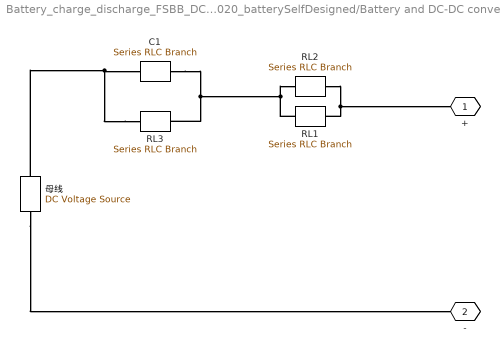
== system Battery_charge_discharge_FSBB_DCDC_r2020_batterySelfDesigned/Battery and DC-DC converter/Subsystem/lithium ion cell (2-RC equivalent circuit model, isothermal)10 ==
  C1 : powerlib/Elements/Series RLC Branch  LConnTagsString=__new0  RConnTagsString=__new0  BranchType=C  Resistance=5  Inductance=1e-3  SetiL0=off  InitialCurrent=0  Capacitance=193  Setx0=off  InitialVoltage=80  Measurements=None
  RL1 : powerlib/Elements/Series RLC Branch  LConnTagsString=__new0  RConnTagsString=__new0  BranchType=R  Resistance=0.86e-3  Inductance=1e-3  SetiL0=off  InitialCurrent=0  Capacitance=1e-6  Setx0=off  InitialVoltage=0  Measurements=None
  RL2 : powerlib/Elements/Series RLC Branch  LConnTagsString=__new0  RConnTagsString=__new0  BranchType=R  Resistance=0.78e-3  Inductance=1e-3  SetiL0=off  InitialCurrent=0  Capacitance=1e-6  Setx0=off  InitialVoltage=0  Measurements=None
  RL3 : powerlib/Elements/Series RLC Branch  LConnTagsString=__new0  RConnTagsString=__new0  BranchType=R  Resistance=0.78e-3  Inductance=1e-3  SetiL0=off  InitialCurrent=0  Capacitance=1e-6  Setx0=off  InitialVoltage=0  Measurements=None
  "母线  " : powerlib/Electrical Sources/DC Voltage Source  Amplitude=3.2  Measurements=None
  + : PMIOPort  Tag=PMCPort  Side=Left
  - : PMIOPort  Tag=PMCPort  Port=2  Side=Right
  connections:
  RL3/LConn1 -- "母线  "/RConn1 -- C1/LConn1
  "母线  "/LConn1 -- -/RConn1
  RL2/RConn1 -- RL1/RConn1 -- +/RConn1
  RL2/LConn1 -- RL1/LConn1 -- RL3/RConn1 -- C1/RConn1

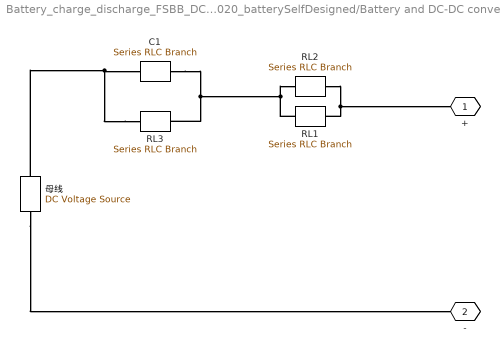
== system Battery_charge_discharge_FSBB_DCDC_r2020_batterySelfDesigned/Battery and DC-DC converter/Subsystem/lithium ion cell (2-RC equivalent circuit model, isothermal)11 ==
  C1 : powerlib/Elements/Series RLC Branch  LConnTagsString=__new0  RConnTagsString=__new0  BranchType=C  Resistance=5  Inductance=1e-3  SetiL0=off  InitialCurrent=0  Capacitance=193  Setx0=off  InitialVoltage=80  Measurements=None
  RL1 : powerlib/Elements/Series RLC Branch  LConnTagsString=__new0  RConnTagsString=__new0  BranchType=R  Resistance=0.86e-3  Inductance=1e-3  SetiL0=off  InitialCurrent=0  Capacitance=1e-6  Setx0=off  InitialVoltage=0  Measurements=None
  RL2 : powerlib/Elements/Series RLC Branch  LConnTagsString=__new0  RConnTagsString=__new0  BranchType=R  Resistance=0.78e-3  Inductance=1e-3  SetiL0=off  InitialCurrent=0  Capacitance=1e-6  Setx0=off  InitialVoltage=0  Measurements=None
  RL3 : powerlib/Elements/Series RLC Branch  LConnTagsString=__new0  RConnTagsString=__new0  BranchType=R  Resistance=0.78e-3  Inductance=1e-3  SetiL0=off  InitialCurrent=0  Capacitance=1e-6  Setx0=off  InitialVoltage=0  Measurements=None
  "母线  " : powerlib/Electrical Sources/DC Voltage Source  Amplitude=3.2  Measurements=None
  + : PMIOPort  Tag=PMCPort  Side=Left
  - : PMIOPort  Tag=PMCPort  Port=2  Side=Right
  connections:
  RL3/LConn1 -- "母线  "/RConn1 -- C1/LConn1
  "母线  "/LConn1 -- -/RConn1
  RL2/RConn1 -- RL1/RConn1 -- +/RConn1
  RL2/LConn1 -- RL1/LConn1 -- RL3/RConn1 -- C1/RConn1

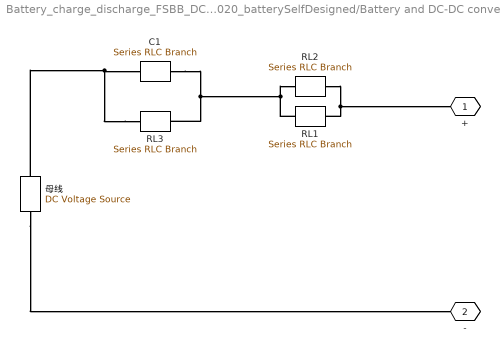
== system Battery_charge_discharge_FSBB_DCDC_r2020_batterySelfDesigned/Battery and DC-DC converter/Subsystem/lithium ion cell (2-RC equivalent circuit model, isothermal)12 ==
  C1 : powerlib/Elements/Series RLC Branch  LConnTagsString=__new0  RConnTagsString=__new0  BranchType=C  Resistance=5  Inductance=1e-3  SetiL0=off  InitialCurrent=0  Capacitance=193  Setx0=off  InitialVoltage=80  Measurements=None
  RL1 : powerlib/Elements/Series RLC Branch  LConnTagsString=__new0  RConnTagsString=__new0  BranchType=R  Resistance=0.86e-3  Inductance=1e-3  SetiL0=off  InitialCurrent=0  Capacitance=1e-6  Setx0=off  InitialVoltage=0  Measurements=None
  RL2 : powerlib/Elements/Series RLC Branch  LConnTagsString=__new0  RConnTagsString=__new0  BranchType=R  Resistance=0.78e-3  Inductance=1e-3  SetiL0=off  InitialCurrent=0  Capacitance=1e-6  Setx0=off  InitialVoltage=0  Measurements=None
  RL3 : powerlib/Elements/Series RLC Branch  LConnTagsString=__new0  RConnTagsString=__new0  BranchType=R  Resistance=0.78e-3  Inductance=1e-3  SetiL0=off  InitialCurrent=0  Capacitance=1e-6  Setx0=off  InitialVoltage=0  Measurements=None
  "母线  " : powerlib/Electrical Sources/DC Voltage Source  Amplitude=3.2  Measurements=None
  + : PMIOPort  Tag=PMCPort  Side=Left
  - : PMIOPort  Tag=PMCPort  Port=2  Side=Right
  connections:
  RL3/LConn1 -- "母线  "/RConn1 -- C1/LConn1
  "母线  "/LConn1 -- -/RConn1
  RL2/RConn1 -- RL1/RConn1 -- +/RConn1
  RL2/LConn1 -- RL1/LConn1 -- RL3/RConn1 -- C1/RConn1

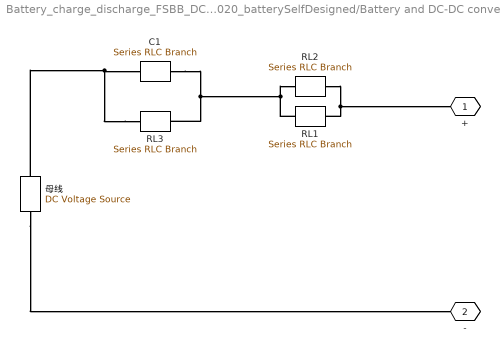
== system Battery_charge_discharge_FSBB_DCDC_r2020_batterySelfDesigned/Battery and DC-DC converter/Subsystem/lithium ion cell (2-RC equivalent circuit model, isothermal)13 ==
  C1 : powerlib/Elements/Series RLC Branch  LConnTagsString=__new0  RConnTagsString=__new0  BranchType=C  Resistance=5  Inductance=1e-3  SetiL0=off  InitialCurrent=0  Capacitance=193  Setx0=off  InitialVoltage=80  Measurements=None
  RL1 : powerlib/Elements/Series RLC Branch  LConnTagsString=__new0  RConnTagsString=__new0  BranchType=R  Resistance=0.86e-3  Inductance=1e-3  SetiL0=off  InitialCurrent=0  Capacitance=1e-6  Setx0=off  InitialVoltage=0  Measurements=None
  RL2 : powerlib/Elements/Series RLC Branch  LConnTagsString=__new0  RConnTagsString=__new0  BranchType=R  Resistance=0.78e-3  Inductance=1e-3  SetiL0=off  InitialCurrent=0  Capacitance=1e-6  Setx0=off  InitialVoltage=0  Measurements=None
  RL3 : powerlib/Elements/Series RLC Branch  LConnTagsString=__new0  RConnTagsString=__new0  BranchType=R  Resistance=0.78e-3  Inductance=1e-3  SetiL0=off  InitialCurrent=0  Capacitance=1e-6  Setx0=off  InitialVoltage=0  Measurements=None
  "母线  " : powerlib/Electrical Sources/DC Voltage Source  Amplitude=3.2  Measurements=None
  + : PMIOPort  Tag=PMCPort  Side=Left
  - : PMIOPort  Tag=PMCPort  Port=2  Side=Right
  connections:
  RL3/LConn1 -- "母线  "/RConn1 -- C1/LConn1
  "母线  "/LConn1 -- -/RConn1
  RL2/RConn1 -- RL1/RConn1 -- +/RConn1
  RL2/LConn1 -- RL1/LConn1 -- RL3/RConn1 -- C1/RConn1

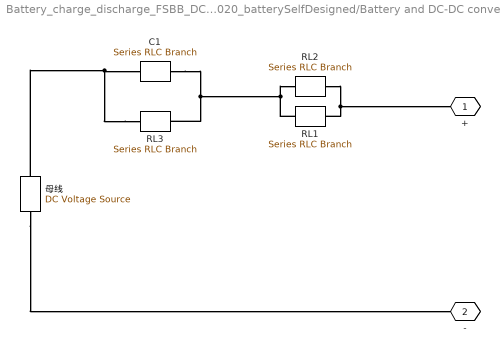
== system Battery_charge_discharge_FSBB_DCDC_r2020_batterySelfDesigned/Battery and DC-DC converter/Subsystem/lithium ion cell (2-RC equivalent circuit model, isothermal)14 ==
  C1 : powerlib/Elements/Series RLC Branch  LConnTagsString=__new0  RConnTagsString=__new0  BranchType=C  Resistance=5  Inductance=1e-3  SetiL0=off  InitialCurrent=0  Capacitance=193  Setx0=off  InitialVoltage=80  Measurements=None
  RL1 : powerlib/Elements/Series RLC Branch  LConnTagsString=__new0  RConnTagsString=__new0  BranchType=R  Resistance=0.86e-3  Inductance=1e-3  SetiL0=off  InitialCurrent=0  Capacitance=1e-6  Setx0=off  InitialVoltage=0  Measurements=None
  RL2 : powerlib/Elements/Series RLC Branch  LConnTagsString=__new0  RConnTagsString=__new0  BranchType=R  Resistance=0.78e-3  Inductance=1e-3  SetiL0=off  InitialCurrent=0  Capacitance=1e-6  Setx0=off  InitialVoltage=0  Measurements=None
  RL3 : powerlib/Elements/Series RLC Branch  LConnTagsString=__new0  RConnTagsString=__new0  BranchType=R  Resistance=0.78e-3  Inductance=1e-3  SetiL0=off  InitialCurrent=0  Capacitance=1e-6  Setx0=off  InitialVoltage=0  Measurements=None
  "母线  " : powerlib/Electrical Sources/DC Voltage Source  Amplitude=3.2  Measurements=None
  + : PMIOPort  Tag=PMCPort  Side=Left
  - : PMIOPort  Tag=PMCPort  Port=2  Side=Right
  connections:
  RL3/LConn1 -- "母线  "/RConn1 -- C1/LConn1
  "母线  "/LConn1 -- -/RConn1
  RL2/RConn1 -- RL1/RConn1 -- +/RConn1
  RL2/LConn1 -- RL1/LConn1 -- RL3/RConn1 -- C1/RConn1

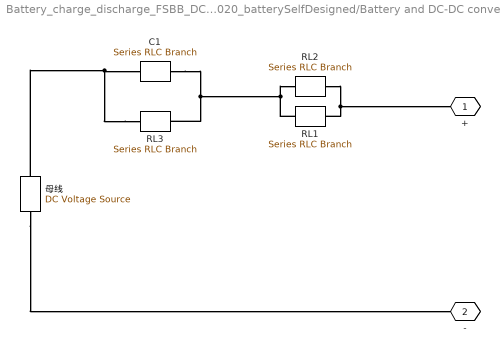
== system Battery_charge_discharge_FSBB_DCDC_r2020_batterySelfDesigned/Battery and DC-DC converter/Subsystem/lithium ion cell (2-RC equivalent circuit model, isothermal)15 ==
  C1 : powerlib/Elements/Series RLC Branch  LConnTagsString=__new0  RConnTagsString=__new0  BranchType=C  Resistance=5  Inductance=1e-3  SetiL0=off  InitialCurrent=0  Capacitance=193  Setx0=off  InitialVoltage=80  Measurements=None
  RL1 : powerlib/Elements/Series RLC Branch  LConnTagsString=__new0  RConnTagsString=__new0  BranchType=R  Resistance=0.86e-3  Inductance=1e-3  SetiL0=off  InitialCurrent=0  Capacitance=1e-6  Setx0=off  InitialVoltage=0  Measurements=None
  RL2 : powerlib/Elements/Series RLC Branch  LConnTagsString=__new0  RConnTagsString=__new0  BranchType=R  Resistance=0.78e-3  Inductance=1e-3  SetiL0=off  InitialCurrent=0  Capacitance=1e-6  Setx0=off  InitialVoltage=0  Measurements=None
  RL3 : powerlib/Elements/Series RLC Branch  LConnTagsString=__new0  RConnTagsString=__new0  BranchType=R  Resistance=0.78e-3  Inductance=1e-3  SetiL0=off  InitialCurrent=0  Capacitance=1e-6  Setx0=off  InitialVoltage=0  Measurements=None
  "母线  " : powerlib/Electrical Sources/DC Voltage Source  Amplitude=3.2  Measurements=None
  + : PMIOPort  Tag=PMCPort  Side=Left
  - : PMIOPort  Tag=PMCPort  Port=2  Side=Right
  connections:
  RL3/LConn1 -- "母线  "/RConn1 -- C1/LConn1
  "母线  "/LConn1 -- -/RConn1
  RL2/RConn1 -- RL1/RConn1 -- +/RConn1
  RL2/LConn1 -- RL1/LConn1 -- RL3/RConn1 -- C1/RConn1

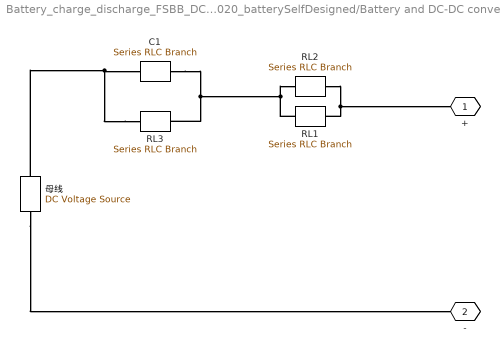
== system Battery_charge_discharge_FSBB_DCDC_r2020_batterySelfDesigned/Battery and DC-DC converter/Subsystem/lithium ion cell (2-RC equivalent circuit model, isothermal)16 ==
  C1 : powerlib/Elements/Series RLC Branch  LConnTagsString=__new0  RConnTagsString=__new0  BranchType=C  Resistance=5  Inductance=1e-3  SetiL0=off  InitialCurrent=0  Capacitance=193  Setx0=off  InitialVoltage=80  Measurements=None
  RL1 : powerlib/Elements/Series RLC Branch  LConnTagsString=__new0  RConnTagsString=__new0  BranchType=R  Resistance=0.86e-3  Inductance=1e-3  SetiL0=off  InitialCurrent=0  Capacitance=1e-6  Setx0=off  InitialVoltage=0  Measurements=None
  RL2 : powerlib/Elements/Series RLC Branch  LConnTagsString=__new0  RConnTagsString=__new0  BranchType=R  Resistance=0.78e-3  Inductance=1e-3  SetiL0=off  InitialCurrent=0  Capacitance=1e-6  Setx0=off  InitialVoltage=0  Measurements=None
  RL3 : powerlib/Elements/Series RLC Branch  LConnTagsString=__new0  RConnTagsString=__new0  BranchType=R  Resistance=0.78e-3  Inductance=1e-3  SetiL0=off  InitialCurrent=0  Capacitance=1e-6  Setx0=off  InitialVoltage=0  Measurements=None
  "母线  " : powerlib/Electrical Sources/DC Voltage Source  Amplitude=3.2  Measurements=None
  + : PMIOPort  Tag=PMCPort  Side=Left
  - : PMIOPort  Tag=PMCPort  Port=2  Side=Right
  connections:
  RL3/LConn1 -- "母线  "/RConn1 -- C1/LConn1
  "母线  "/LConn1 -- -/RConn1
  RL2/RConn1 -- RL1/RConn1 -- +/RConn1
  RL2/LConn1 -- RL1/LConn1 -- RL3/RConn1 -- C1/RConn1
